simulink model "Close_Loop_Model_Simulink"  (R2019a)
settings: Solver=VariableStepAuto  StartTime=0.0  StopTime=400  RelTol=1e-3
values from neighbouring files (symbols this model uses):
  c = 1.0791e-5    (= 1.0791e-05)    [Initial_Parameters.m]
  J = J_motor + (J_robot)*(1/G)^2    (= 3.96043)    [Initial_Parameters.m]
  ke = 50.68*60/(2*pi*1000)    (= 0.483958350954)    [Initial_Parameters.m]
  km = 0.415    [Initial_Parameters.m]
  L = 4.8*1e-3    (= 0.0048)    [Initial_Parameters.m]
  R = 9.65    [Initial_Parameters.m]
libraries: simulink x1
settings Model: Creator=sp_ja  LastModifiedBy=sp_ja

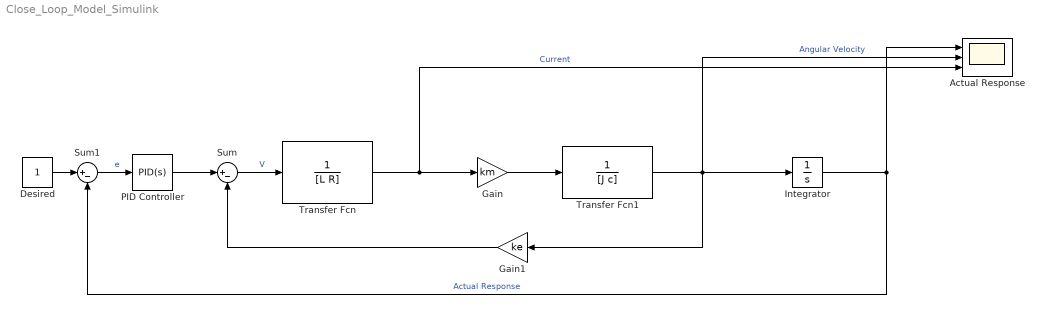
== system Close_Loop_Model_Simulink ==
  Actual Response : Scope  NumInputPorts=3
  Desired : Constant
  "Gain " : Gain  Gain=km
  "Gain1 " : Gain  Gain=ke
  "Integrator " : Integrator
  PID Controller : simulink/Continuous/PID Controller  Controller=PID  Form=Parallel  TimeDomain=Continuous-time  SampleTime=-1  IntegratorMethod=Forward Euler  FilterMethod=Forward Euler  ControllerParametersSource=internal  P=0.173  I=0.00077  D=7.819  UseFilter=on  N=9.89340066287468  TunerSelectOption=Transfer Function Based (PID Tuner App)  InitialConditionSource=internal  InitialConditionForIntegrator=0  InitialConditionForFilter=0  DifferentiatorICPrevScaledInput=0  ExternalReset=none  TrackingMode=off  Kt=1  LimitOutput=off  UpperSaturationLimit=inf  LowerSaturationLimit=-inf  LinearizeAsGain=on  AntiWindupMode=none  Kb=1  POutMin=[]  POutMax=[]  IOutMin=[]  IOutMax=[]  DOutMin=[]  DOutMax=[]  NOutMin=[]  NOutMax=[]  SumOutMin=[]  SumOutMax=[]  SaturationOutMin=[]  SaturationOutMax=[]  PParamMin=[]  PParamMax=[]  IParamMin=[]  IParamMax=[]  DParamMin=[]  DParamMax=[]  NParamMin=[]  NParamMax=[]  KbParamMin=[]  KbParamMax=[]  KtParamMin=[]  KtParamMax=[]  KbOutMin=[]  KbOutMax=[]  KtOutMin=[]  KtOutMax=[]  IntegratorOutMin=[]  IntegratorOutMax=[]  FilterOutMin=[]  FilterOutMax=[]  SumI1OutMin=[]  SumI1OutMax=[]  SumI2OutMin=[]  SumI2OutMax=[]  SumI3OutMin=[]  SumI3OutMax=[]  SumI4OutMin=[]  SumI4OutMax=[]  SumDOutMin=[]  SumDOutMax=[]  DifferentiatorOutMin=[]  DifferentiatorOutMax=[]  FilterDiffOutCoefMin=[]  FilterDiffOutCoefMax=[]  ReciprocalOutMin=[]  ReciprocalOutMax=[]  SumDenOutMin=[]  SumDenOutMax=[]  SumNumOutMin=[]  SumNumOutMax=[]  DivideOutMin=[]  DivideOutMax=[]  IntegratorContinuousStateAttributes=''  IntegratorStateMustResolveToSignalObject=off  IntegratorRTWStateStorageClass=Auto  FilterContinuousStateAttributes=''  FilterStateMustResolveToSignalObject=off  FilterRTWStateStorageClass=Auto  ParallelPVariant=InternalParameters  IdealPVariant=Disabled  IVariant=InternalParameters  DVariant=InternalParameters  IntegratorVariant=Continuous  SatVariant=Disabled  AWVariant=Passthrough  PCopyVariant=Disabled  TRVariant=Disabled  FdbkBlocksVariant=Forward  IdealPFdbkVariant=Disabled  SatFdbkVariant=Disabled  DerivativeFilterVariant=ContFilter  NVariant=InternalParameters  NCopyVariant=Disabled  FilterICVariant=InternalICsFilter  IntegratorICVariant=InternalICs  ExternalResetVariant=Disabled  TRSumVariant=Passthrough  SumFdbkVariant=Disabled  SumVariant=Sum_PID
  Sum : Sum  Inputs=|+-
  Sum1 : Sum  Inputs=|+-
  "Transfer Fcn " : TransferFcn  Denominator=[L R]
  "Transfer Fcn1 " : TransferFcn  Denominator=[J c]
  wires:
  "Gain1 "/1 -> Sum/2
  PID Controller/1 -> Sum/1
  "Gain "/1 -> "Transfer Fcn1 "/1
  "Integrator "/1 -> Actual Response/1, Sum1/2  "Actual Response"
  "Transfer Fcn1 "/1 -> Actual Response/2, "Integrator "/1, "Gain1 "/1  "Angular Velocity"
  "Transfer Fcn "/1 -> Actual Response/3, "Gain "/1  "Current"
  Sum/1 -> "Transfer Fcn "/1  "V"
  Sum1/1 -> PID Controller/1  "e"
  Desired/1 -> Sum1/1
